simulink model "bee2_complex_corr"  (Simulink 7.0)
settings: Solver=ode45  StartTime=0.0  StopTime=10.0  RelTol=1e-3
undefined symbols (not defined in the file or in its folder): BEE2_usr
libraries: xbsIndex_r4 x279, xps_library x61, casper_library_misc x18
(part 2 of 4)

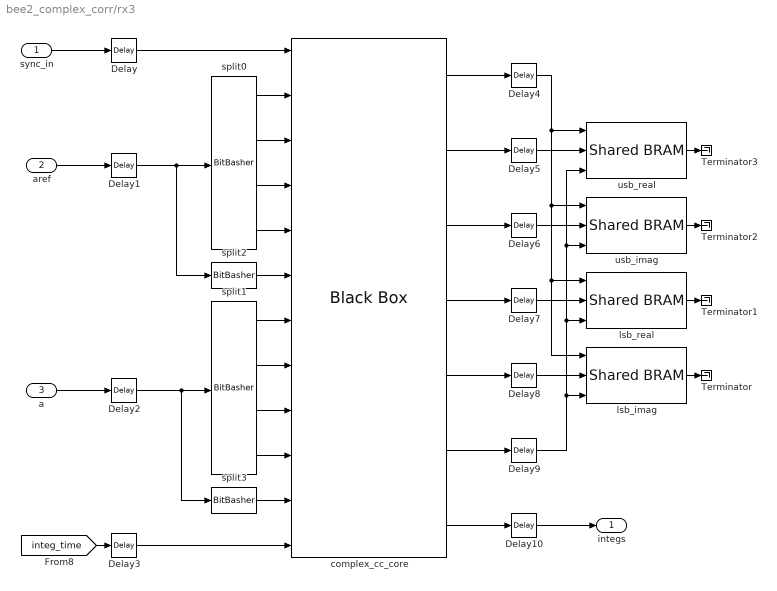
== system bee2_complex_corr/rx3 ==
  sync_in : Inport  OutDataType=sfix(16)  OutScaling=2^0
  aref : Inport  Port=2  OutDataType=sfix(16)  OutScaling=2^0
  a : Inport  Port=3  OutDataType=sfix(16)  OutScaling=2^0
  Delay{,1..10} (11 alike) : xbsIndex_r4/Delay  en=off  latency=1  dbl_ovrd=off  reg_retiming=off  block_type=delay
  Terminator{,1..3} (4 alike) : Terminator
  complex_cc_core : xbsIndex_r4/Black Box  init_code=complex_cc_core_config  sim_method=Inactive  block_type=blackbox2
      settings: infoedit="Incorporates black box HDL and simulation model into a System Generator design.<P><P>You must supply a Black Box with certain information about the HDL component you would like to bring into System Generator. This information is provided through a Matlab function.<P><P>When \"Simulation mode\" is set to \"Inactive\", you will typically want to provide a separate simulation model by using a Simulation Multiplexer.<P>When \"Simulation mode\" is set to \"External co-simulator\", you must include a ModelSim block in the design."  block_version=10.1.3
  lsb_imag : xps_library/Shared BRAM  Tag=xps:bram  SystemSampleTime=-1  arith_type="Signed  (2's comp)"  addr_width=11  data_width=32  data_bin_pt=0  init_vals=0  sample_rate=1
      link override bee2_complex_corr_0x0_func_real_data_out: arith_type="Signed  (2's comp)"
      link override bee2_complex_corr_corr00_func_real_data_out: arith_type="Signed  (2's comp)"
      link override bee2_complex_corr_corr01_func_real_data_out: arith_type="Signed  (2's comp)"
      link override bee2_complex_corr_rx3_lsb_imag_data_out: arith_type="Signed  (2's comp)"
      link override convert_din: arith_type="Signed  (2's comp)"
      link override correlator_2bit_bee2_output_corr0_data_out: arith_type=Unsigned
      link override correlator_2bit_bee2_x2_output_corr01_data_out: arith_type=Unsigned
      link override correlator_2bit_bee2_x2_output_corr0_data_out: arith_type=Unsigned
      link override correlator_2bit_ibob_output_corr0_data_out: arith_type=Unsigned
      link override cross_correlator_test_corr_out_data_out: arith_type="Signed  (2's comp)"
      link override cross_correlator_test_input_data1_data_out: arith_type=Unsigned
      link override dbe_xaui_corr_corr_func_data_out: arith_type="Signed  (2's comp)"
      link override dbe_xaui_corr_new_xaui_summer_summer_output_corr_data_out: arith_type="Signed  (2's comp)"
      link override dbe_xaui_corr_xaui_summer_summer_output_corr_data_out: arith_type="Signed  (2's comp)"
      link override mem/sim_data_in: arith_type="Signed  (2's comp)"
  lsb_real : xps_library/Shared BRAM  Tag=xps:bram  SystemSampleTime=-1  arith_type="Signed  (2's comp)"  addr_width=11  data_width=32  data_bin_pt=0  init_vals=0  sample_rate=1
      link override bee2_complex_corr_0x0_func_real_data_out: arith_type="Signed  (2's comp)"
      link override bee2_complex_corr_corr00_func_real_data_out: arith_type="Signed  (2's comp)"
      link override bee2_complex_corr_corr01_func_real_data_out: arith_type="Signed  (2's comp)"
      link override bee2_complex_corr_rx3_lsb_real_data_out: arith_type="Signed  (2's comp)"
      link override convert_din: arith_type="Signed  (2's comp)"
      link override correlator_2bit_bee2_output_corr0_data_out: arith_type=Unsigned
      link override correlator_2bit_bee2_x2_output_corr01_data_out: arith_type=Unsigned
      link override correlator_2bit_bee2_x2_output_corr0_data_out: arith_type=Unsigned
      link override correlator_2bit_ibob_output_corr0_data_out: arith_type=Unsigned
      link override cross_correlator_test_corr_out_data_out: arith_type="Signed  (2's comp)"
      link override cross_correlator_test_input_data1_data_out: arith_type=Unsigned
      link override dbe_xaui_corr_corr_func_data_out: arith_type="Signed  (2's comp)"
      link override dbe_xaui_corr_new_xaui_summer_summer_output_corr_data_out: arith_type="Signed  (2's comp)"
      link override dbe_xaui_corr_xaui_summer_summer_output_corr_data_out: arith_type="Signed  (2's comp)"
      link override mem/sim_data_in: arith_type="Signed  (2's comp)"
  split0 : xbsIndex_r4/BitBasher  bitexpr=|  display_expr=off  sr_1=1  arith_type1=Unsigned  bin_pt1=0  sr_2=2  arith_type2=Unsigned  bin_pt2=0  sr_3=3  arith_type3=Unsigned  bin_pt3=0  sr_4=4  arith_type4=Unsigned  bin_pt4=0  dbl_ovrd=off  block_type=bitbasher
      | <html><head><meta name="qrichtext" content="1" /><style type="text/css">
      | p, li { white-space: pre-wrap; }
      | </style></head><body style=" font-family:'MS Shell Dlg 2'; font-size:8.25pt; font-weight:400; font-style:normal;">
      | <p style=" margin-top:0px; margin-bottom:0px; margin-left:0px; margin-right:0px; -qt-block-indent:0; text-indent:0px; font-size:8pt;">r0={a[8:7]}<br />i0={a[6:5]}<br /><span style=" font-family:'MS Shell Dlg';">r1={a[4:3]}<br />i1={a[2:1]}</span></p></body></html>
      settings: block_version=10.1.3
  split1 : xbsIndex_r4/BitBasher  bitexpr=|  display_expr=off  sr_1=1  arith_type1=Unsigned  bin_pt1=0  sr_2=2  arith_type2=Unsigned  bin_pt2=0  sr_3=3  arith_type3=Unsigned  bin_pt3=0  sr_4=4  arith_type4=Unsigned  bin_pt4=0  dbl_ovrd=off  block_type=bitbasher
      | <html><head><meta name="qrichtext" content="1" /><style type="text/css">
      | p, li { white-space: pre-wrap; }
      | </style></head><body style=" font-family:'MS Shell Dlg 2'; font-size:8.25pt; font-weight:400; font-style:normal;">
      | <p style=" margin-top:0px; margin-bottom:0px; margin-left:0px; margin-right:0px; -qt-block-indent:0; text-indent:0px; font-size:8pt;">r0={a[8:7]}<br />i0={a[6:5]}<br /><span style=" font-family:'MS Shell Dlg';">r1={a[4:3]}<br />i1={a[2:1]}</span></p></body></html>
      settings: block_version=10.1.3
  split2 : xbsIndex_r4/BitBasher  bitexpr=|  display_expr=off  sr_1=1  arith_type1=Unsigned  bin_pt1=0  sr_2=2  arith_type2=Unsigned  bin_pt2=0  sr_3=3  arith_type3=Unsigned  bin_pt3=0  sr_4=4  arith_type4=Unsigned  bin_pt4=0  dbl_ovrd=off  block_type=bitbasher
      | <html><head><meta name="qrichtext" content="1" /><style type="text/css">
      | p, li { white-space: pre-wrap; }
      | </style></head><body style=" font-family:'MS Shell Dlg 2'; font-size:8.25pt; font-weight:400; font-style:normal;">
      | <p style=" margin-top:0px; margin-bottom:0px; margin-left:0px; margin-right:0px; -qt-block-indent:0; text-indent:0px; font-size:8pt;"><span style=" font-family:'MS Shell Dlg';">w={a[0]}</span></p></body></html>
      settings: block_version=10.1.3
  split3 : xbsIndex_r4/BitBasher  bitexpr=|  display_expr=off  sr_1=1  arith_type1=Unsigned  bin_pt1=0  sr_2=2  arith_type2=Unsigned  bin_pt2=0  sr_3=3  arith_type3=Unsigned  bin_pt3=0  sr_4=4  arith_type4=Unsigned  bin_pt4=0  dbl_ovrd=off  block_type=bitbasher
      | <html><head><meta name="qrichtext" content="1" /><style type="text/css">
      | p, li { white-space: pre-wrap; }
      | </style></head><body style=" font-family:'MS Shell Dlg 2'; font-size:8.25pt; font-weight:400; font-style:normal;">
      | <p style=" margin-top:0px; margin-bottom:0px; margin-left:0px; margin-right:0px; -qt-block-indent:0; text-indent:0px; font-size:8pt;"><span style=" font-family:'MS Shell Dlg';">w={a[0]}</span></p></body></html>
      settings: block_version=10.1.3
  usb_imag : xps_library/Shared BRAM  Tag=xps:bram  SystemSampleTime=-1  arith_type="Signed  (2's comp)"  addr_width=11  data_width=32  data_bin_pt=0  init_vals=0  sample_rate=1
      link override bee2_complex_corr_0x0_func_real_data_out: arith_type="Signed  (2's comp)"
      link override bee2_complex_corr_corr00_func_real_data_out: arith_type="Signed  (2's comp)"
      link override bee2_complex_corr_corr01_func_real_data_out: arith_type="Signed  (2's comp)"
      link override bee2_complex_corr_rx3_usb_imag_data_out: arith_type="Signed  (2's comp)"
      link override convert_din: arith_type="Signed  (2's comp)"
      link override correlator_2bit_bee2_output_corr0_data_out: arith_type=Unsigned
      link override correlator_2bit_bee2_x2_output_corr01_data_out: arith_type=Unsigned
      link override correlator_2bit_bee2_x2_output_corr0_data_out: arith_type=Unsigned
      link override correlator_2bit_ibob_output_corr0_data_out: arith_type=Unsigned
      link override cross_correlator_test_corr_out_data_out: arith_type="Signed  (2's comp)"
      link override cross_correlator_test_input_data1_data_out: arith_type=Unsigned
      link override dbe_xaui_corr_corr_func_data_out: arith_type="Signed  (2's comp)"
      link override dbe_xaui_corr_new_xaui_summer_summer_output_corr_data_out: arith_type="Signed  (2's comp)"
      link override dbe_xaui_corr_xaui_summer_summer_output_corr_data_out: arith_type="Signed  (2's comp)"
      link override mem/sim_data_in: arith_type="Signed  (2's comp)"
  usb_real : xps_library/Shared BRAM  Tag=xps:bram  SystemSampleTime=-1  arith_type="Signed  (2's comp)"  addr_width=11  data_width=32  data_bin_pt=0  init_vals=0  sample_rate=1
      link override bee2_complex_corr_0x0_func_real_data_out: arith_type="Signed  (2's comp)"
      link override bee2_complex_corr_corr00_func_real_data_out: arith_type="Signed  (2's comp)"
      link override bee2_complex_corr_corr01_func_real_data_out: arith_type="Signed  (2's comp)"
      link override bee2_complex_corr_rx3_usb_real_data_out: arith_type="Signed  (2's comp)"
      link override convert_din: arith_type="Signed  (2's comp)"
      link override correlator_2bit_bee2_output_corr0_data_out: arith_type=Unsigned
      link override correlator_2bit_bee2_x2_output_corr01_data_out: arith_type=Unsigned
      link override correlator_2bit_bee2_x2_output_corr0_data_out: arith_type=Unsigned
      link override correlator_2bit_ibob_output_corr0_data_out: arith_type=Unsigned
      link override cross_correlator_test_corr_out_data_out: arith_type="Signed  (2's comp)"
      link override cross_correlator_test_input_data1_data_out: arith_type=Unsigned
      link override dbe_xaui_corr_corr_func_data_out: arith_type="Signed  (2's comp)"
      link override dbe_xaui_corr_new_xaui_summer_summer_output_corr_data_out: arith_type="Signed  (2's comp)"
      link override dbe_xaui_corr_xaui_summer_summer_output_corr_data_out: arith_type="Signed  (2's comp)"
      link override mem/sim_data_in: arith_type="Signed  (2's comp)"
  integs : Outport  OutDataType=sfix(16)  OutScaling=2^0
  wires:
  [integ_time] -> Delay3/1
  a/1 -> Delay2/1
  aref/1 -> Delay1/1
  split0/4 -> complex_cc_core/5
  split0/3 -> complex_cc_core/4
  split0/2 -> complex_cc_core/3
  split0/1 -> complex_cc_core/2
  sync_in/1 -> Delay/1
  complex_cc_core/1 -> Delay4/1
  complex_cc_core/2 -> Delay5/1
  complex_cc_core/3 -> Delay6/1
  complex_cc_core/4 -> Delay7/1
  complex_cc_core/5 -> Delay8/1
  Delay/1 -> complex_cc_core/1
  Delay1/1 -> split0/1, split2/1
  Delay2/1 -> split1/1, split3/1
  Delay7/1 -> lsb_real/2
  Delay8/1 -> lsb_imag/2
  Delay10/1 -> integs/1
  complex_cc_core/6 -> Delay9/1
  complex_cc_core/7 -> Delay10/1
  Delay5/1 -> usb_real/2
  Delay6/1 -> usb_imag/2
  Delay3/1 -> complex_cc_core/12
  split2/1 -> complex_cc_core/6
  split1/1 -> complex_cc_core/7
  split1/2 -> complex_cc_core/8
  split1/3 -> complex_cc_core/9
  split1/4 -> complex_cc_core/10
  split3/1 -> complex_cc_core/11
  Delay4/1 -> usb_real/1, usb_imag/1, lsb_imag/1, lsb_real/1
  Delay9/1 -> usb_real/3, usb_imag/3, lsb_real/3, lsb_imag/3
  lsb_imag/1 -> Terminator/1
  lsb_real/1 -> Terminator1/1
  usb_imag/1 -> Terminator2/1
  usb_real/1 -> Terminator3/1

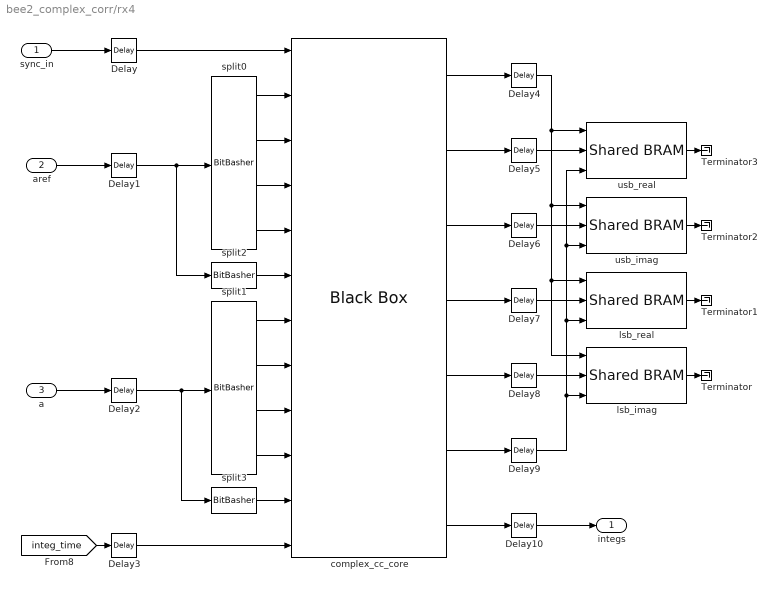
== system bee2_complex_corr/rx4 ==
  sync_in : Inport  OutDataType=sfix(16)  OutScaling=2^0
  aref : Inport  Port=2  OutDataType=sfix(16)  OutScaling=2^0
  a : Inport  Port=3  OutDataType=sfix(16)  OutScaling=2^0
  Delay{,1..10} (11 alike) : xbsIndex_r4/Delay  en=off  latency=1  dbl_ovrd=off  reg_retiming=off  block_type=delay
  Terminator{,1..3} (4 alike) : Terminator
  complex_cc_core : xbsIndex_r4/Black Box  init_code=complex_cc_core_config  sim_method=Inactive  block_type=blackbox2
      settings: infoedit="Incorporates black box HDL and simulation model into a System Generator design.<P><P>You must supply a Black Box with certain information about the HDL component you would like to bring into System Generator. This information is provided through a Matlab function.<P><P>When \"Simulation mode\" is set to \"Inactive\", you will typically want to provide a separate simulation model by using a Simulation Multiplexer.<P>When \"Simulation mode\" is set to \"External co-simulator\", you must include a ModelSim block in the design."  block_version=10.1.3
  lsb_imag : xps_library/Shared BRAM  Tag=xps:bram  SystemSampleTime=-1  arith_type="Signed  (2's comp)"  addr_width=11  data_width=32  data_bin_pt=0  init_vals=0  sample_rate=1
      link override bee2_complex_corr_0x0_func_real_data_out: arith_type="Signed  (2's comp)"
      link override bee2_complex_corr_corr00_func_real_data_out: arith_type="Signed  (2's comp)"
      link override bee2_complex_corr_corr01_func_real_data_out: arith_type="Signed  (2's comp)"
      link override bee2_complex_corr_rx4_lsb_imag_data_out: arith_type="Signed  (2's comp)"
      link override convert_din: arith_type="Signed  (2's comp)"
      link override correlator_2bit_bee2_output_corr0_data_out: arith_type=Unsigned
      link override correlator_2bit_bee2_x2_output_corr01_data_out: arith_type=Unsigned
      link override correlator_2bit_bee2_x2_output_corr0_data_out: arith_type=Unsigned
      link override correlator_2bit_ibob_output_corr0_data_out: arith_type=Unsigned
      link override cross_correlator_test_corr_out_data_out: arith_type="Signed  (2's comp)"
      link override cross_correlator_test_input_data1_data_out: arith_type=Unsigned
      link override dbe_xaui_corr_corr_func_data_out: arith_type="Signed  (2's comp)"
      link override dbe_xaui_corr_new_xaui_summer_summer_output_corr_data_out: arith_type="Signed  (2's comp)"
      link override dbe_xaui_corr_xaui_summer_summer_output_corr_data_out: arith_type="Signed  (2's comp)"
      link override mem/sim_data_in: arith_type="Signed  (2's comp)"
  lsb_real : xps_library/Shared BRAM  Tag=xps:bram  SystemSampleTime=-1  arith_type="Signed  (2's comp)"  addr_width=11  data_width=32  data_bin_pt=0  init_vals=0  sample_rate=1
      link override bee2_complex_corr_0x0_func_real_data_out: arith_type="Signed  (2's comp)"
      link override bee2_complex_corr_corr00_func_real_data_out: arith_type="Signed  (2's comp)"
      link override bee2_complex_corr_corr01_func_real_data_out: arith_type="Signed  (2's comp)"
      link override bee2_complex_corr_rx4_lsb_real_data_out: arith_type="Signed  (2's comp)"
      link override convert_din: arith_type="Signed  (2's comp)"
      link override correlator_2bit_bee2_output_corr0_data_out: arith_type=Unsigned
      link override correlator_2bit_bee2_x2_output_corr01_data_out: arith_type=Unsigned
      link override correlator_2bit_bee2_x2_output_corr0_data_out: arith_type=Unsigned
      link override correlator_2bit_ibob_output_corr0_data_out: arith_type=Unsigned
      link override cross_correlator_test_corr_out_data_out: arith_type="Signed  (2's comp)"
      link override cross_correlator_test_input_data1_data_out: arith_type=Unsigned
      link override dbe_xaui_corr_corr_func_data_out: arith_type="Signed  (2's comp)"
      link override dbe_xaui_corr_new_xaui_summer_summer_output_corr_data_out: arith_type="Signed  (2's comp)"
      link override dbe_xaui_corr_xaui_summer_summer_output_corr_data_out: arith_type="Signed  (2's comp)"
      link override mem/sim_data_in: arith_type="Signed  (2's comp)"
  split0 : xbsIndex_r4/BitBasher  bitexpr=|  display_expr=off  sr_1=1  arith_type1=Unsigned  bin_pt1=0  sr_2=2  arith_type2=Unsigned  bin_pt2=0  sr_3=3  arith_type3=Unsigned  bin_pt3=0  sr_4=4  arith_type4=Unsigned  bin_pt4=0  dbl_ovrd=off  block_type=bitbasher
      | <html><head><meta name="qrichtext" content="1" /><style type="text/css">
      | p, li { white-space: pre-wrap; }
      | </style></head><body style=" font-family:'MS Shell Dlg 2'; font-size:8.25pt; font-weight:400; font-style:normal;">
      | <p style=" margin-top:0px; margin-bottom:0px; margin-left:0px; margin-right:0px; -qt-block-indent:0; text-indent:0px; font-size:8pt;">r0={a[8:7]}<br />i0={a[6:5]}<br /><span style=" font-family:'MS Shell Dlg';">r1={a[4:3]}<br />i1={a[2:1]}</span></p></body></html>
      settings: block_version=10.1.3
  split1 : xbsIndex_r4/BitBasher  bitexpr=|  display_expr=off  sr_1=1  arith_type1=Unsigned  bin_pt1=0  sr_2=2  arith_type2=Unsigned  bin_pt2=0  sr_3=3  arith_type3=Unsigned  bin_pt3=0  sr_4=4  arith_type4=Unsigned  bin_pt4=0  dbl_ovrd=off  block_type=bitbasher
      | <html><head><meta name="qrichtext" content="1" /><style type="text/css">
      | p, li { white-space: pre-wrap; }
      | </style></head><body style=" font-family:'MS Shell Dlg 2'; font-size:8.25pt; font-weight:400; font-style:normal;">
      | <p style=" margin-top:0px; margin-bottom:0px; margin-left:0px; margin-right:0px; -qt-block-indent:0; text-indent:0px; font-size:8pt;">r0={a[8:7]}<br />i0={a[6:5]}<br /><span style=" font-family:'MS Shell Dlg';">r1={a[4:3]}<br />i1={a[2:1]}</span></p></body></html>
      settings: block_version=10.1.3
  split2 : xbsIndex_r4/BitBasher  bitexpr=|  display_expr=off  sr_1=1  arith_type1=Unsigned  bin_pt1=0  sr_2=2  arith_type2=Unsigned  bin_pt2=0  sr_3=3  arith_type3=Unsigned  bin_pt3=0  sr_4=4  arith_type4=Unsigned  bin_pt4=0  dbl_ovrd=off  block_type=bitbasher
      | <html><head><meta name="qrichtext" content="1" /><style type="text/css">
      | p, li { white-space: pre-wrap; }
      | </style></head><body style=" font-family:'MS Shell Dlg 2'; font-size:8.25pt; font-weight:400; font-style:normal;">
      | <p style=" margin-top:0px; margin-bottom:0px; margin-left:0px; margin-right:0px; -qt-block-indent:0; text-indent:0px; font-size:8pt;"><span style=" font-family:'MS Shell Dlg';">w={a[0]}</span></p></body></html>
      settings: block_version=10.1.3
  split3 : xbsIndex_r4/BitBasher  bitexpr=|  display_expr=off  sr_1=1  arith_type1=Unsigned  bin_pt1=0  sr_2=2  arith_type2=Unsigned  bin_pt2=0  sr_3=3  arith_type3=Unsigned  bin_pt3=0  sr_4=4  arith_type4=Unsigned  bin_pt4=0  dbl_ovrd=off  block_type=bitbasher
      | <html><head><meta name="qrichtext" content="1" /><style type="text/css">
      | p, li { white-space: pre-wrap; }
      | </style></head><body style=" font-family:'MS Shell Dlg 2'; font-size:8.25pt; font-weight:400; font-style:normal;">
      | <p style=" margin-top:0px; margin-bottom:0px; margin-left:0px; margin-right:0px; -qt-block-indent:0; text-indent:0px; font-size:8pt;"><span style=" font-family:'MS Shell Dlg';">w={a[0]}</span></p></body></html>
      settings: block_version=10.1.3
  usb_imag : xps_library/Shared BRAM  Tag=xps:bram  SystemSampleTime=-1  arith_type="Signed  (2's comp)"  addr_width=11  data_width=32  data_bin_pt=0  init_vals=0  sample_rate=1
      link override bee2_complex_corr_0x0_func_real_data_out: arith_type="Signed  (2's comp)"
      link override bee2_complex_corr_corr00_func_real_data_out: arith_type="Signed  (2's comp)"
      link override bee2_complex_corr_corr01_func_real_data_out: arith_type="Signed  (2's comp)"
      link override bee2_complex_corr_rx4_usb_imag_data_out: arith_type="Signed  (2's comp)"
      link override convert_din: arith_type="Signed  (2's comp)"
      link override correlator_2bit_bee2_output_corr0_data_out: arith_type=Unsigned
      link override correlator_2bit_bee2_x2_output_corr01_data_out: arith_type=Unsigned
      link override correlator_2bit_bee2_x2_output_corr0_data_out: arith_type=Unsigned
      link override correlator_2bit_ibob_output_corr0_data_out: arith_type=Unsigned
      link override cross_correlator_test_corr_out_data_out: arith_type="Signed  (2's comp)"
      link override cross_correlator_test_input_data1_data_out: arith_type=Unsigned
      link override dbe_xaui_corr_corr_func_data_out: arith_type="Signed  (2's comp)"
      link override dbe_xaui_corr_new_xaui_summer_summer_output_corr_data_out: arith_type="Signed  (2's comp)"
      link override dbe_xaui_corr_xaui_summer_summer_output_corr_data_out: arith_type="Signed  (2's comp)"
      link override mem/sim_data_in: arith_type="Signed  (2's comp)"
  usb_real : xps_library/Shared BRAM  Tag=xps:bram  SystemSampleTime=-1  arith_type="Signed  (2's comp)"  addr_width=11  data_width=32  data_bin_pt=0  init_vals=0  sample_rate=1
      link override bee2_complex_corr_0x0_func_real_data_out: arith_type="Signed  (2's comp)"
      link override bee2_complex_corr_corr00_func_real_data_out: arith_type="Signed  (2's comp)"
      link override bee2_complex_corr_corr01_func_real_data_out: arith_type="Signed  (2's comp)"
      link override bee2_complex_corr_rx4_usb_real_data_out: arith_type="Signed  (2's comp)"
      link override convert_din: arith_type="Signed  (2's comp)"
      link override correlator_2bit_bee2_output_corr0_data_out: arith_type=Unsigned
      link override correlator_2bit_bee2_x2_output_corr01_data_out: arith_type=Unsigned
      link override correlator_2bit_bee2_x2_output_corr0_data_out: arith_type=Unsigned
      link override correlator_2bit_ibob_output_corr0_data_out: arith_type=Unsigned
      link override cross_correlator_test_corr_out_data_out: arith_type="Signed  (2's comp)"
      link override cross_correlator_test_input_data1_data_out: arith_type=Unsigned
      link override dbe_xaui_corr_corr_func_data_out: arith_type="Signed  (2's comp)"
      link override dbe_xaui_corr_new_xaui_summer_summer_output_corr_data_out: arith_type="Signed  (2's comp)"
      link override dbe_xaui_corr_xaui_summer_summer_output_corr_data_out: arith_type="Signed  (2's comp)"
      link override mem/sim_data_in: arith_type="Signed  (2's comp)"
  integs : Outport  OutDataType=sfix(16)  OutScaling=2^0
  wires:
  [integ_time] -> Delay3/1
  a/1 -> Delay2/1
  aref/1 -> Delay1/1
  split0/4 -> complex_cc_core/5
  split0/3 -> complex_cc_core/4
  split0/2 -> complex_cc_core/3
  split0/1 -> complex_cc_core/2
  sync_in/1 -> Delay/1
  complex_cc_core/1 -> Delay4/1
  complex_cc_core/2 -> Delay5/1
  complex_cc_core/3 -> Delay6/1
  complex_cc_core/4 -> Delay7/1
  complex_cc_core/5 -> Delay8/1
  Delay/1 -> complex_cc_core/1
  Delay1/1 -> split0/1, split2/1
  Delay2/1 -> split1/1, split3/1
  Delay7/1 -> lsb_real/2
  Delay8/1 -> lsb_imag/2
  Delay10/1 -> integs/1
  complex_cc_core/6 -> Delay9/1
  complex_cc_core/7 -> Delay10/1
  Delay5/1 -> usb_real/2
  Delay6/1 -> usb_imag/2
  Delay3/1 -> complex_cc_core/12
  split2/1 -> complex_cc_core/6
  split1/1 -> complex_cc_core/7
  split1/2 -> complex_cc_core/8
  split1/3 -> complex_cc_core/9
  split1/4 -> complex_cc_core/10
  split3/1 -> complex_cc_core/11
  Delay4/1 -> usb_real/1, usb_imag/1, lsb_imag/1, lsb_real/1
  Delay9/1 -> usb_real/3, usb_imag/3, lsb_real/3, lsb_imag/3
  lsb_imag/1 -> Terminator/1
  lsb_real/1 -> Terminator1/1
  usb_imag/1 -> Terminator2/1
  usb_real/1 -> Terminator3/1

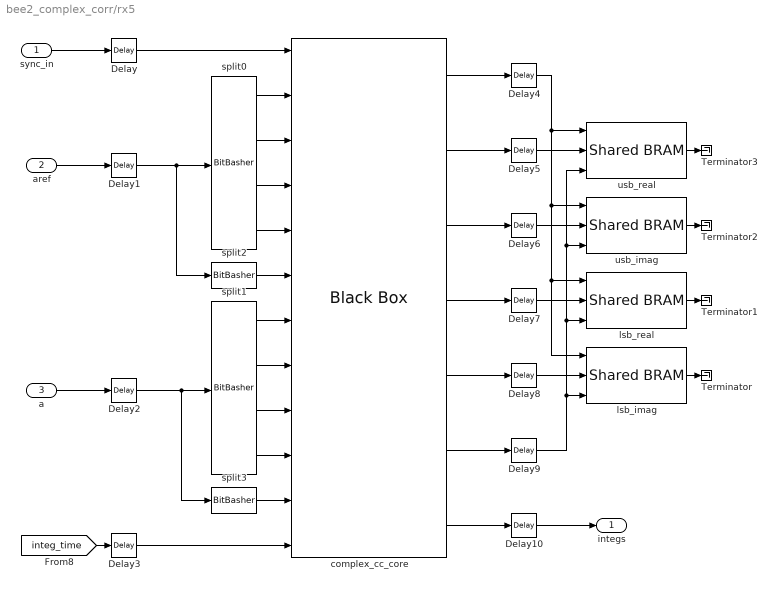
== system bee2_complex_corr/rx5 ==
  sync_in : Inport  OutDataType=sfix(16)  OutScaling=2^0
  aref : Inport  Port=2  OutDataType=sfix(16)  OutScaling=2^0
  a : Inport  Port=3  OutDataType=sfix(16)  OutScaling=2^0
  Delay{,1..10} (11 alike) : xbsIndex_r4/Delay  en=off  latency=1  dbl_ovrd=off  reg_retiming=off  block_type=delay
  Terminator{,1..3} (4 alike) : Terminator
  complex_cc_core : xbsIndex_r4/Black Box  init_code=complex_cc_core_config  sim_method=Inactive  block_type=blackbox2
      settings: infoedit="Incorporates black box HDL and simulation model into a System Generator design.<P><P>You must supply a Black Box with certain information about the HDL component you would like to bring into System Generator. This information is provided through a Matlab function.<P><P>When \"Simulation mode\" is set to \"Inactive\", you will typically want to provide a separate simulation model by using a Simulation Multiplexer.<P>When \"Simulation mode\" is set to \"External co-simulator\", you must include a ModelSim block in the design."  block_version=10.1.3
  lsb_imag : xps_library/Shared BRAM  Tag=xps:bram  SystemSampleTime=-1  arith_type="Signed  (2's comp)"  addr_width=11  data_width=32  data_bin_pt=0  init_vals=0  sample_rate=1
      link override bee2_complex_corr_0x0_func_real_data_out: arith_type="Signed  (2's comp)"
      link override bee2_complex_corr_corr00_func_real_data_out: arith_type="Signed  (2's comp)"
      link override bee2_complex_corr_corr01_func_real_data_out: arith_type="Signed  (2's comp)"
      link override bee2_complex_corr_rx5_lsb_imag_data_out: arith_type="Signed  (2's comp)"
      link override convert_din: arith_type="Signed  (2's comp)"
      link override correlator_2bit_bee2_output_corr0_data_out: arith_type=Unsigned
      link override correlator_2bit_bee2_x2_output_corr01_data_out: arith_type=Unsigned
      link override correlator_2bit_bee2_x2_output_corr0_data_out: arith_type=Unsigned
      link override correlator_2bit_ibob_output_corr0_data_out: arith_type=Unsigned
      link override cross_correlator_test_corr_out_data_out: arith_type="Signed  (2's comp)"
      link override cross_correlator_test_input_data1_data_out: arith_type=Unsigned
      link override dbe_xaui_corr_corr_func_data_out: arith_type="Signed  (2's comp)"
      link override dbe_xaui_corr_new_xaui_summer_summer_output_corr_data_out: arith_type="Signed  (2's comp)"
      link override dbe_xaui_corr_xaui_summer_summer_output_corr_data_out: arith_type="Signed  (2's comp)"
      link override mem/sim_data_in: arith_type="Signed  (2's comp)"
  lsb_real : xps_library/Shared BRAM  Tag=xps:bram  SystemSampleTime=-1  arith_type="Signed  (2's comp)"  addr_width=11  data_width=32  data_bin_pt=0  init_vals=0  sample_rate=1
      link override bee2_complex_corr_0x0_func_real_data_out: arith_type="Signed  (2's comp)"
      link override bee2_complex_corr_corr00_func_real_data_out: arith_type="Signed  (2's comp)"
      link override bee2_complex_corr_corr01_func_real_data_out: arith_type="Signed  (2's comp)"
      link override bee2_complex_corr_rx5_lsb_real_data_out: arith_type="Signed  (2's comp)"
      link override convert_din: arith_type="Signed  (2's comp)"
      link override correlator_2bit_bee2_output_corr0_data_out: arith_type=Unsigned
      link override correlator_2bit_bee2_x2_output_corr01_data_out: arith_type=Unsigned
      link override correlator_2bit_bee2_x2_output_corr0_data_out: arith_type=Unsigned
      link override correlator_2bit_ibob_output_corr0_data_out: arith_type=Unsigned
      link override cross_correlator_test_corr_out_data_out: arith_type="Signed  (2's comp)"
      link override cross_correlator_test_input_data1_data_out: arith_type=Unsigned
      link override dbe_xaui_corr_corr_func_data_out: arith_type="Signed  (2's comp)"
      link override dbe_xaui_corr_new_xaui_summer_summer_output_corr_data_out: arith_type="Signed  (2's comp)"
      link override dbe_xaui_corr_xaui_summer_summer_output_corr_data_out: arith_type="Signed  (2's comp)"
      link override mem/sim_data_in: arith_type="Signed  (2's comp)"
  split0 : xbsIndex_r4/BitBasher  bitexpr=|  display_expr=off  sr_1=1  arith_type1=Unsigned  bin_pt1=0  sr_2=2  arith_type2=Unsigned  bin_pt2=0  sr_3=3  arith_type3=Unsigned  bin_pt3=0  sr_4=4  arith_type4=Unsigned  bin_pt4=0  dbl_ovrd=off  block_type=bitbasher
      | <html><head><meta name="qrichtext" content="1" /><style type="text/css">
      | p, li { white-space: pre-wrap; }
      | </style></head><body style=" font-family:'MS Shell Dlg 2'; font-size:8.25pt; font-weight:400; font-style:normal;">
      | <p style=" margin-top:0px; margin-bottom:0px; margin-left:0px; margin-right:0px; -qt-block-indent:0; text-indent:0px; font-size:8pt;">r0={a[8:7]}<br />i0={a[6:5]}<br /><span style=" font-family:'MS Shell Dlg';">r1={a[4:3]}<br />i1={a[2:1]}</span></p></body></html>
      settings: block_version=10.1.3
  split1 : xbsIndex_r4/BitBasher  bitexpr=|  display_expr=off  sr_1=1  arith_type1=Unsigned  bin_pt1=0  sr_2=2  arith_type2=Unsigned  bin_pt2=0  sr_3=3  arith_type3=Unsigned  bin_pt3=0  sr_4=4  arith_type4=Unsigned  bin_pt4=0  dbl_ovrd=off  block_type=bitbasher
      | <html><head><meta name="qrichtext" content="1" /><style type="text/css">
      | p, li { white-space: pre-wrap; }
      | </style></head><body style=" font-family:'MS Shell Dlg 2'; font-size:8.25pt; font-weight:400; font-style:normal;">
      | <p style=" margin-top:0px; margin-bottom:0px; margin-left:0px; margin-right:0px; -qt-block-indent:0; text-indent:0px; font-size:8pt;">r0={a[8:7]}<br />i0={a[6:5]}<br /><span style=" font-family:'MS Shell Dlg';">r1={a[4:3]}<br />i1={a[2:1]}</span></p></body></html>
      settings: block_version=10.1.3
  split2 : xbsIndex_r4/BitBasher  bitexpr=|  display_expr=off  sr_1=1  arith_type1=Unsigned  bin_pt1=0  sr_2=2  arith_type2=Unsigned  bin_pt2=0  sr_3=3  arith_type3=Unsigned  bin_pt3=0  sr_4=4  arith_type4=Unsigned  bin_pt4=0  dbl_ovrd=off  block_type=bitbasher
      | <html><head><meta name="qrichtext" content="1" /><style type="text/css">
      | p, li { white-space: pre-wrap; }
      | </style></head><body style=" font-family:'MS Shell Dlg 2'; font-size:8.25pt; font-weight:400; font-style:normal;">
      | <p style=" margin-top:0px; margin-bottom:0px; margin-left:0px; margin-right:0px; -qt-block-indent:0; text-indent:0px; font-size:8pt;"><span style=" font-family:'MS Shell Dlg';">w={a[0]}</span></p></body></html>
      settings: block_version=10.1.3
  split3 : xbsIndex_r4/BitBasher  bitexpr=|  display_expr=off  sr_1=1  arith_type1=Unsigned  bin_pt1=0  sr_2=2  arith_type2=Unsigned  bin_pt2=0  sr_3=3  arith_type3=Unsigned  bin_pt3=0  sr_4=4  arith_type4=Unsigned  bin_pt4=0  dbl_ovrd=off  block_type=bitbasher
      | <html><head><meta name="qrichtext" content="1" /><style type="text/css">
      | p, li { white-space: pre-wrap; }
      | </style></head><body style=" font-family:'MS Shell Dlg 2'; font-size:8.25pt; font-weight:400; font-style:normal;">
      | <p style=" margin-top:0px; margin-bottom:0px; margin-left:0px; margin-right:0px; -qt-block-indent:0; text-indent:0px; font-size:8pt;"><span style=" font-family:'MS Shell Dlg';">w={a[0]}</span></p></body></html>
      settings: block_version=10.1.3
  usb_imag : xps_library/Shared BRAM  Tag=xps:bram  SystemSampleTime=-1  arith_type="Signed  (2's comp)"  addr_width=11  data_width=32  data_bin_pt=0  init_vals=0  sample_rate=1
      link override bee2_complex_corr_0x0_func_real_data_out: arith_type="Signed  (2's comp)"
      link override bee2_complex_corr_corr00_func_real_data_out: arith_type="Signed  (2's comp)"
      link override bee2_complex_corr_corr01_func_real_data_out: arith_type="Signed  (2's comp)"
      link override bee2_complex_corr_rx5_usb_imag_data_out: arith_type="Signed  (2's comp)"
      link override convert_din: arith_type="Signed  (2's comp)"
      link override correlator_2bit_bee2_output_corr0_data_out: arith_type=Unsigned
      link override correlator_2bit_bee2_x2_output_corr01_data_out: arith_type=Unsigned
      link override correlator_2bit_bee2_x2_output_corr0_data_out: arith_type=Unsigned
      link override correlator_2bit_ibob_output_corr0_data_out: arith_type=Unsigned
      link override cross_correlator_test_corr_out_data_out: arith_type="Signed  (2's comp)"
      link override cross_correlator_test_input_data1_data_out: arith_type=Unsigned
      link override dbe_xaui_corr_corr_func_data_out: arith_type="Signed  (2's comp)"
      link override dbe_xaui_corr_new_xaui_summer_summer_output_corr_data_out: arith_type="Signed  (2's comp)"
      link override dbe_xaui_corr_xaui_summer_summer_output_corr_data_out: arith_type="Signed  (2's comp)"
      link override mem/sim_data_in: arith_type="Signed  (2's comp)"
  usb_real : xps_library/Shared BRAM  Tag=xps:bram  SystemSampleTime=-1  arith_type="Signed  (2's comp)"  addr_width=11  data_width=32  data_bin_pt=0  init_vals=0  sample_rate=1
      link override bee2_complex_corr_0x0_func_real_data_out: arith_type="Signed  (2's comp)"
      link override bee2_complex_corr_corr00_func_real_data_out: arith_type="Signed  (2's comp)"
      link override bee2_complex_corr_corr01_func_real_data_out: arith_type="Signed  (2's comp)"
      link override bee2_complex_corr_rx5_usb_real_data_out: arith_type="Signed  (2's comp)"
      link override convert_din: arith_type="Signed  (2's comp)"
      link override correlator_2bit_bee2_output_corr0_data_out: arith_type=Unsigned
      link override correlator_2bit_bee2_x2_output_corr01_data_out: arith_type=Unsigned
      link override correlator_2bit_bee2_x2_output_corr0_data_out: arith_type=Unsigned
      link override correlator_2bit_ibob_output_corr0_data_out: arith_type=Unsigned
      link override cross_correlator_test_corr_out_data_out: arith_type="Signed  (2's comp)"
      link override cross_correlator_test_input_data1_data_out: arith_type=Unsigned
      link override dbe_xaui_corr_corr_func_data_out: arith_type="Signed  (2's comp)"
      link override dbe_xaui_corr_new_xaui_summer_summer_output_corr_data_out: arith_type="Signed  (2's comp)"
      link override dbe_xaui_corr_xaui_summer_summer_output_corr_data_out: arith_type="Signed  (2's comp)"
      link override mem/sim_data_in: arith_type="Signed  (2's comp)"
  integs : Outport  OutDataType=sfix(16)  OutScaling=2^0
  wires:
  [integ_time] -> Delay3/1
  a/1 -> Delay2/1
  aref/1 -> Delay1/1
  split0/4 -> complex_cc_core/5
  split0/3 -> complex_cc_core/4
  split0/2 -> complex_cc_core/3
  split0/1 -> complex_cc_core/2
  sync_in/1 -> Delay/1
  complex_cc_core/1 -> Delay4/1
  complex_cc_core/2 -> Delay5/1
  complex_cc_core/3 -> Delay6/1
  complex_cc_core/4 -> Delay7/1
  complex_cc_core/5 -> Delay8/1
  Delay/1 -> complex_cc_core/1
  Delay1/1 -> split0/1, split2/1
  Delay2/1 -> split1/1, split3/1
  Delay7/1 -> lsb_real/2
  Delay8/1 -> lsb_imag/2
  Delay10/1 -> integs/1
  complex_cc_core/6 -> Delay9/1
  complex_cc_core/7 -> Delay10/1
  Delay5/1 -> usb_real/2
  Delay6/1 -> usb_imag/2
  Delay3/1 -> complex_cc_core/12
  split2/1 -> complex_cc_core/6
  split1/1 -> complex_cc_core/7
  split1/2 -> complex_cc_core/8
  split1/3 -> complex_cc_core/9
  split1/4 -> complex_cc_core/10
  split3/1 -> complex_cc_core/11
  Delay4/1 -> usb_real/1, usb_imag/1, lsb_imag/1, lsb_real/1
  Delay9/1 -> usb_real/3, usb_imag/3, lsb_real/3, lsb_imag/3
  lsb_imag/1 -> Terminator/1
  lsb_real/1 -> Terminator1/1
  usb_imag/1 -> Terminator2/1
  usb_real/1 -> Terminator3/1

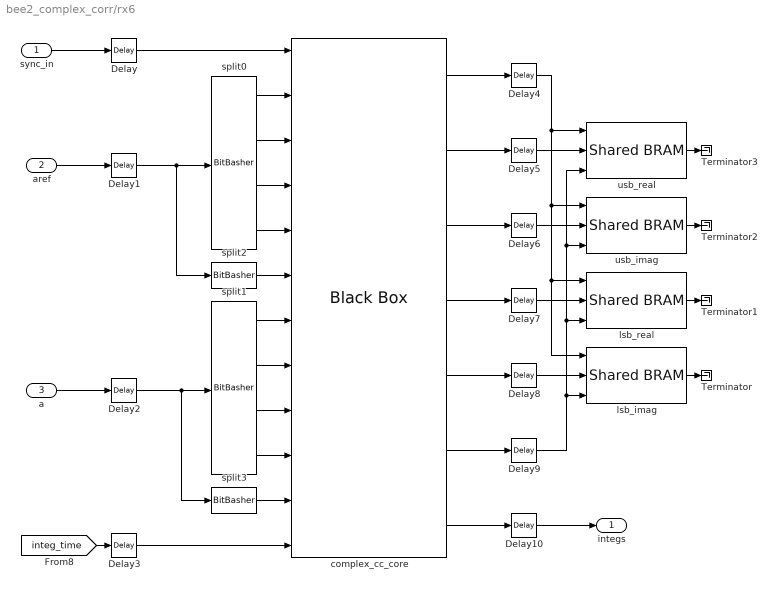
== system bee2_complex_corr/rx6 ==
  sync_in : Inport  OutDataType=sfix(16)  OutScaling=2^0
  aref : Inport  Port=2  OutDataType=sfix(16)  OutScaling=2^0
  a : Inport  Port=3  OutDataType=sfix(16)  OutScaling=2^0
  Delay{,1..10} (11 alike) : xbsIndex_r4/Delay  en=off  latency=1  dbl_ovrd=off  reg_retiming=off  block_type=delay
  Terminator{,1..3} (4 alike) : Terminator
  complex_cc_core : xbsIndex_r4/Black Box  init_code=complex_cc_core_config  sim_method=Inactive  block_type=blackbox2
      settings: infoedit="Incorporates black box HDL and simulation model into a System Generator design.<P><P>You must supply a Black Box with certain information about the HDL component you would like to bring into System Generator. This information is provided through a Matlab function.<P><P>When \"Simulation mode\" is set to \"Inactive\", you will typically want to provide a separate simulation model by using a Simulation Multiplexer.<P>When \"Simulation mode\" is set to \"External co-simulator\", you must include a ModelSim block in the design."  block_version=10.1.3
  lsb_imag : xps_library/Shared BRAM  Tag=xps:bram  SystemSampleTime=-1  arith_type="Signed  (2's comp)"  addr_width=11  data_width=32  data_bin_pt=0  init_vals=0  sample_rate=1
      link override bee2_complex_corr_0x0_func_real_data_out: arith_type="Signed  (2's comp)"
      link override bee2_complex_corr_corr00_func_real_data_out: arith_type="Signed  (2's comp)"
      link override bee2_complex_corr_corr01_func_real_data_out: arith_type="Signed  (2's comp)"
      link override bee2_complex_corr_rx6_lsb_imag_data_out: arith_type="Signed  (2's comp)"
      link override convert_din: arith_type="Signed  (2's comp)"
      link override correlator_2bit_bee2_output_corr0_data_out: arith_type=Unsigned
      link override correlator_2bit_bee2_x2_output_corr01_data_out: arith_type=Unsigned
      link override correlator_2bit_bee2_x2_output_corr0_data_out: arith_type=Unsigned
      link override correlator_2bit_ibob_output_corr0_data_out: arith_type=Unsigned
      link override cross_correlator_test_corr_out_data_out: arith_type="Signed  (2's comp)"
      link override cross_correlator_test_input_data1_data_out: arith_type=Unsigned
      link override dbe_xaui_corr_corr_func_data_out: arith_type="Signed  (2's comp)"
      link override dbe_xaui_corr_new_xaui_summer_summer_output_corr_data_out: arith_type="Signed  (2's comp)"
      link override dbe_xaui_corr_xaui_summer_summer_output_corr_data_out: arith_type="Signed  (2's comp)"
      link override mem/sim_data_in: arith_type="Signed  (2's comp)"
  lsb_real : xps_library/Shared BRAM  Tag=xps:bram  SystemSampleTime=-1  arith_type="Signed  (2's comp)"  addr_width=11  data_width=32  data_bin_pt=0  init_vals=0  sample_rate=1
      link override bee2_complex_corr_0x0_func_real_data_out: arith_type="Signed  (2's comp)"
      link override bee2_complex_corr_corr00_func_real_data_out: arith_type="Signed  (2's comp)"
      link override bee2_complex_corr_corr01_func_real_data_out: arith_type="Signed  (2's comp)"
      link override bee2_complex_corr_rx6_lsb_real_data_out: arith_type="Signed  (2's comp)"
      link override convert_din: arith_type="Signed  (2's comp)"
      link override correlator_2bit_bee2_output_corr0_data_out: arith_type=Unsigned
      link override correlator_2bit_bee2_x2_output_corr01_data_out: arith_type=Unsigned
      link override correlator_2bit_bee2_x2_output_corr0_data_out: arith_type=Unsigned
      link override correlator_2bit_ibob_output_corr0_data_out: arith_type=Unsigned
      link override cross_correlator_test_corr_out_data_out: arith_type="Signed  (2's comp)"
      link override cross_correlator_test_input_data1_data_out: arith_type=Unsigned
      link override dbe_xaui_corr_corr_func_data_out: arith_type="Signed  (2's comp)"
      link override dbe_xaui_corr_new_xaui_summer_summer_output_corr_data_out: arith_type="Signed  (2's comp)"
      link override dbe_xaui_corr_xaui_summer_summer_output_corr_data_out: arith_type="Signed  (2's comp)"
      link override mem/sim_data_in: arith_type="Signed  (2's comp)"
  split0 : xbsIndex_r4/BitBasher  bitexpr=|  display_expr=off  sr_1=1  arith_type1=Unsigned  bin_pt1=0  sr_2=2  arith_type2=Unsigned  bin_pt2=0  sr_3=3  arith_type3=Unsigned  bin_pt3=0  sr_4=4  arith_type4=Unsigned  bin_pt4=0  dbl_ovrd=off  block_type=bitbasher
      | <html><head><meta name="qrichtext" content="1" /><style type="text/css">
      | p, li { white-space: pre-wrap; }
      | </style></head><body style=" font-family:'MS Shell Dlg 2'; font-size:8.25pt; font-weight:400; font-style:normal;">
      | <p style=" margin-top:0px; margin-bottom:0px; margin-left:0px; margin-right:0px; -qt-block-indent:0; text-indent:0px; font-size:8pt;">r0={a[8:7]}<br />i0={a[6:5]}<br /><span style=" font-family:'MS Shell Dlg';">r1={a[4:3]}<br />i1={a[2:1]}</span></p></body></html>
      settings: block_version=10.1.3
  split1 : xbsIndex_r4/BitBasher  bitexpr=|  display_expr=off  sr_1=1  arith_type1=Unsigned  bin_pt1=0  sr_2=2  arith_type2=Unsigned  bin_pt2=0  sr_3=3  arith_type3=Unsigned  bin_pt3=0  sr_4=4  arith_type4=Unsigned  bin_pt4=0  dbl_ovrd=off  block_type=bitbasher
      | <html><head><meta name="qrichtext" content="1" /><style type="text/css">
      | p, li { white-space: pre-wrap; }
      | </style></head><body style=" font-family:'MS Shell Dlg 2'; font-size:8.25pt; font-weight:400; font-style:normal;">
      | <p style=" margin-top:0px; margin-bottom:0px; margin-left:0px; margin-right:0px; -qt-block-indent:0; text-indent:0px; font-size:8pt;">r0={a[8:7]}<br />i0={a[6:5]}<br /><span style=" font-family:'MS Shell Dlg';">r1={a[4:3]}<br />i1={a[2:1]}</span></p></body></html>
      settings: block_version=10.1.3
  split2 : xbsIndex_r4/BitBasher  bitexpr=|  display_expr=off  sr_1=1  arith_type1=Unsigned  bin_pt1=0  sr_2=2  arith_type2=Unsigned  bin_pt2=0  sr_3=3  arith_type3=Unsigned  bin_pt3=0  sr_4=4  arith_type4=Unsigned  bin_pt4=0  dbl_ovrd=off  block_type=bitbasher
      | <html><head><meta name="qrichtext" content="1" /><style type="text/css">
      | p, li { white-space: pre-wrap; }
      | </style></head><body style=" font-family:'MS Shell Dlg 2'; font-size:8.25pt; font-weight:400; font-style:normal;">
      | <p style=" margin-top:0px; margin-bottom:0px; margin-left:0px; margin-right:0px; -qt-block-indent:0; text-indent:0px; font-size:8pt;"><span style=" font-family:'MS Shell Dlg';">w={a[0]}</span></p></body></html>
      settings: block_version=10.1.3
  split3 : xbsIndex_r4/BitBasher  bitexpr=|  display_expr=off  sr_1=1  arith_type1=Unsigned  bin_pt1=0  sr_2=2  arith_type2=Unsigned  bin_pt2=0  sr_3=3  arith_type3=Unsigned  bin_pt3=0  sr_4=4  arith_type4=Unsigned  bin_pt4=0  dbl_ovrd=off  block_type=bitbasher
      | <html><head><meta name="qrichtext" content="1" /><style type="text/css">
      | p, li { white-space: pre-wrap; }
      | </style></head><body style=" font-family:'MS Shell Dlg 2'; font-size:8.25pt; font-weight:400; font-style:normal;">
      | <p style=" margin-top:0px; margin-bottom:0px; margin-left:0px; margin-right:0px; -qt-block-indent:0; text-indent:0px; font-size:8pt;"><span style=" font-family:'MS Shell Dlg';">w={a[0]}</span></p></body></html>
      settings: block_version=10.1.3
  usb_imag : xps_library/Shared BRAM  Tag=xps:bram  SystemSampleTime=-1  arith_type="Signed  (2's comp)"  addr_width=11  data_width=32  data_bin_pt=0  init_vals=0  sample_rate=1
      link override bee2_complex_corr_0x0_func_real_data_out: arith_type="Signed  (2's comp)"
      link override bee2_complex_corr_corr00_func_real_data_out: arith_type="Signed  (2's comp)"
      link override bee2_complex_corr_corr01_func_real_data_out: arith_type="Signed  (2's comp)"
      link override bee2_complex_corr_rx6_usb_imag_data_out: arith_type="Signed  (2's comp)"
      link override convert_din: arith_type="Signed  (2's comp)"
      link override correlator_2bit_bee2_output_corr0_data_out: arith_type=Unsigned
      link override correlator_2bit_bee2_x2_output_corr01_data_out: arith_type=Unsigned
      link override correlator_2bit_bee2_x2_output_corr0_data_out: arith_type=Unsigned
      link override correlator_2bit_ibob_output_corr0_data_out: arith_type=Unsigned
      link override cross_correlator_test_corr_out_data_out: arith_type="Signed  (2's comp)"
      link override cross_correlator_test_input_data1_data_out: arith_type=Unsigned
      link override dbe_xaui_corr_corr_func_data_out: arith_type="Signed  (2's comp)"
      link override dbe_xaui_corr_new_xaui_summer_summer_output_corr_data_out: arith_type="Signed  (2's comp)"
      link override dbe_xaui_corr_xaui_summer_summer_output_corr_data_out: arith_type="Signed  (2's comp)"
      link override mem/sim_data_in: arith_type="Signed  (2's comp)"
  usb_real : xps_library/Shared BRAM  Tag=xps:bram  SystemSampleTime=-1  arith_type="Signed  (2's comp)"  addr_width=11  data_width=32  data_bin_pt=0  init_vals=0  sample_rate=1
      link override bee2_complex_corr_0x0_func_real_data_out: arith_type="Signed  (2's comp)"
      link override bee2_complex_corr_corr00_func_real_data_out: arith_type="Signed  (2's comp)"
      link override bee2_complex_corr_corr01_func_real_data_out: arith_type="Signed  (2's comp)"
      link override bee2_complex_corr_rx6_usb_real_data_out: arith_type="Signed  (2's comp)"
      link override convert_din: arith_type="Signed  (2's comp)"
      link override correlator_2bit_bee2_output_corr0_data_out: arith_type=Unsigned
      link override correlator_2bit_bee2_x2_output_corr01_data_out: arith_type=Unsigned
      link override correlator_2bit_bee2_x2_output_corr0_data_out: arith_type=Unsigned
      link override correlator_2bit_ibob_output_corr0_data_out: arith_type=Unsigned
      link override cross_correlator_test_corr_out_data_out: arith_type="Signed  (2's comp)"
      link override cross_correlator_test_input_data1_data_out: arith_type=Unsigned
      link override dbe_xaui_corr_corr_func_data_out: arith_type="Signed  (2's comp)"
      link override dbe_xaui_corr_new_xaui_summer_summer_output_corr_data_out: arith_type="Signed  (2's comp)"
      link override dbe_xaui_corr_xaui_summer_summer_output_corr_data_out: arith_type="Signed  (2's comp)"
      link override mem/sim_data_in: arith_type="Signed  (2's comp)"
  integs : Outport  OutDataType=sfix(16)  OutScaling=2^0
  wires:
  [integ_time] -> Delay3/1
  a/1 -> Delay2/1
  aref/1 -> Delay1/1
  split0/4 -> complex_cc_core/5
  split0/3 -> complex_cc_core/4
  split0/2 -> complex_cc_core/3
  split0/1 -> complex_cc_core/2
  sync_in/1 -> Delay/1
  complex_cc_core/1 -> Delay4/1
  complex_cc_core/2 -> Delay5/1
  complex_cc_core/3 -> Delay6/1
  complex_cc_core/4 -> Delay7/1
  complex_cc_core/5 -> Delay8/1
  Delay/1 -> complex_cc_core/1
  Delay1/1 -> split0/1, split2/1
  Delay2/1 -> split1/1, split3/1
  Delay7/1 -> lsb_real/2
  Delay8/1 -> lsb_imag/2
  Delay10/1 -> integs/1
  complex_cc_core/6 -> Delay9/1
  complex_cc_core/7 -> Delay10/1
  Delay5/1 -> usb_real/2
  Delay6/1 -> usb_imag/2
  Delay3/1 -> complex_cc_core/12
  split2/1 -> complex_cc_core/6
  split1/1 -> complex_cc_core/7
  split1/2 -> complex_cc_core/8
  split1/3 -> complex_cc_core/9
  split1/4 -> complex_cc_core/10
  split3/1 -> complex_cc_core/11
  Delay4/1 -> usb_real/1, usb_imag/1, lsb_imag/1, lsb_real/1
  Delay9/1 -> usb_real/3, usb_imag/3, lsb_real/3, lsb_imag/3
  lsb_imag/1 -> Terminator/1
  lsb_real/1 -> Terminator1/1
  usb_imag/1 -> Terminator2/1
  usb_real/1 -> Terminator3/1
